simulink model "ARP_01_lib_TruthTables"  (R2014a)
settings: Solver=ode45  StartTime=0.0  StopTime=10.0  RelTol=1e-3
(part 1 of 2)
settings Model: Creator=Maryam  LastModifiedBy=Maryam

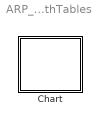
== system ARP_01_lib_TruthTables ==
  Chart : Stateflow chart  TreatAsAtomicUnit=on
